simulink subsystem "Aerodyn"  (R2020b)
settings: Solver=VariableStepAuto  StartTime=0.0  StopTime=10.0  RelTol=1e-3
undefined symbols (not defined in the file or in its folder): Aerodynamics
settings Model: Creator=NicolasS  LastModifiedBy=leifr

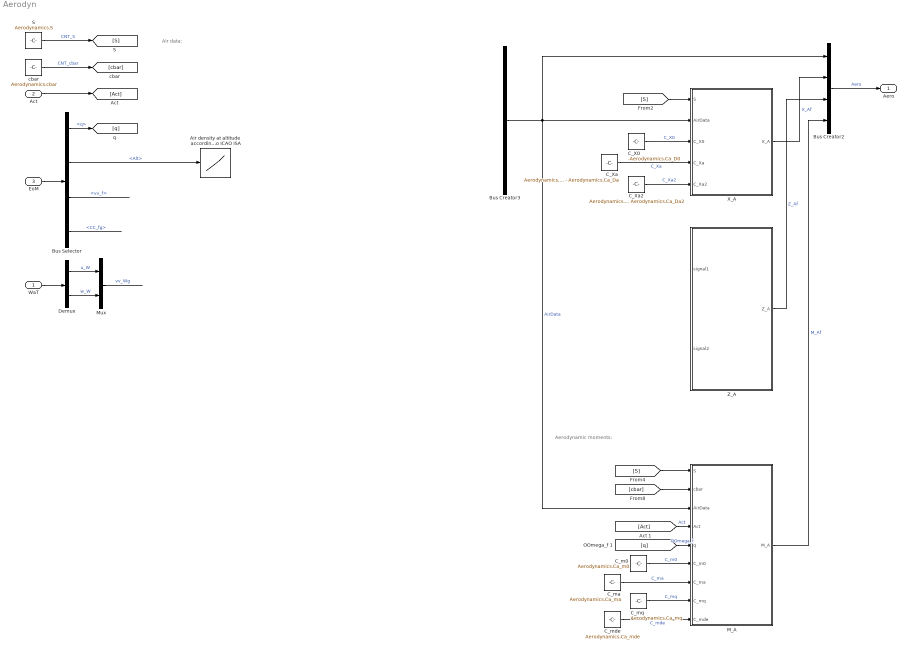
== system Aerodyn ==
  note: Aerodynamic moments:
  note: Air data:
  WaT : Inport
  Act : Inport  Port=2  OutDataTypeStr=Bus: Act
  EoM : Inport  Port=3  OutDataTypeStr=Bus: EoM
  Air density at altitude according to ICAO ISA : Lookup_n-D  NumberOfTableDimensions=1  BreakpointsForDimension1=Aerodynamics.LUT_Alt  Table=Aerodynamics.LUT_rho  ExtrapMethod=Clip  InternalRulePriority=Speed  RndMeth=Simplest  InputSameDT=on
  Bus Creator2 : BusCreator  Inputs=4  OutDataTypeStr=Bus: Aero
  Bus Creator3 : BusCreator  Inputs=5  OutDataTypeStr=Bus: AirData
  Bus Selector : BusSelector  OutputSignals=q,Alt,vv_f,CC.CC_fg
  C_X0 : Constant  Value=-Aerodynamics.Ca_D0  VectorParams1D=off  OutDataTypeStr=double  SampleTime=-1
  C_Xa : Constant  Value=Aerodynamics.Ca_L0 - Aerodynamics.Ca_Da  VectorParams1D=off  OutDataTypeStr=double  SampleTime=-1
  C_Xa2 : Constant  Value=Aerodynamics.Ca_La - Aerodynamics.Ca_Da2  VectorParams1D=off  OutDataTypeStr=double  SampleTime=-1
  C_m0 : Constant  Value=Aerodynamics.Ca_m0  VectorParams1D=off  OutDataTypeStr=double  SampleTime=-1
  C_ma : Constant  Value=Aerodynamics.Ca_ma  VectorParams1D=off  OutDataTypeStr=double  SampleTime=-1
  C_mde : Constant  Value=Aerodynamics.Ca_mde  VectorParams1D=off  OutDataTypeStr=double  SampleTime=-1
  C_mq : Constant  Value=Aerodynamics.Ca_mq  VectorParams1D=off  OutDataTypeStr=double  SampleTime=-1
  Demux : Demux  Outputs=2
  M_A : MATLAB Function  TreatAsAtomicUnit=on
  Mux : Mux  Inputs=2
  S : Constant  Value=Aerodynamics.S  OutDataTypeStr=double  SampleTime=-1
  X_A : MATLAB Function  TreatAsAtomicUnit=on
  Z_A : MATLAB Function  TreatAsAtomicUnit=on
  cbar : Constant  Value=Aerodynamics.cbar  OutDataTypeStr=double  SampleTime=-1
  Aero : Outport  OutDataTypeStr=Bus: Aero
  wires:
  C_m0/1 -> M_A/6(C_m0)  "C_m0"
  Bus Selector/4 -> ?  "<CC_fg>"
  ? -> Bus Creator3/1  "u_Af"
  Bus Creator2/1 -> Aero/1  "Aero"
  C_mde/1 -> M_A/9(C_mde)  "C_mde"
  S/1 -> [S]  "CNT_S"
  C_Xa/1 -> X_A/4(C_Xa)  "C_Xa"
  Bus Creator3/1 -> X_A/2(AirData), M_A/3(AirData), Bus Creator2/1  "AirData"
  EoM/1 -> Bus Selector/1
  M_A/1(M_A) -> Bus Creator2/4  "M_Af"
  Z_A/1(Z_A) -> Bus Creator2/3  "Z_Af"
  ? -> Bus Creator3/2  "w_Af"
  C_ma/1 -> M_A/7(C_ma)  "C_ma"
  C_mq/1 -> M_A/8(C_mq)  "C_mq"
  X_A/1(X_A) -> Bus Creator2/2  "X_Af"
  C_X0/1 -> X_A/3(C_X0)  "C_X0"
  [S] -> M_A/1(S)
  [q] -> M_A/5(q)  "OOmega_f"
  ? -> Bus Creator3/4  "p_dyn"
  [Act] -> M_A/4(Act)  "Act"
  Demux/2 -> Mux/2  "w_W"
  [cbar] -> M_A/2(cbar)
  Bus Selector/2 -> Air density at altitude according to ICAO ISA/1  "<Alt>"
  C_Xa2/1 -> X_A/5(C_Xa2)  "C_Xa2"
  WaT/1 -> Demux/1
  cbar/1 -> [cbar]  "CNT_cbar"
  Bus Selector/1 -> [q]  "<q>"
  Mux/1 -> ?  "vv_Wg"
  Demux/1 -> Mux/1  "u_W"
  Act/1 -> [Act]
  ? -> Bus Creator3/3  "V_A"
  [S] -> X_A/1(S)
  ? -> Bus Creator3/5  "alpha"
  Bus Selector/3 -> ?  "<vv_f>"

== matlab function Aerodyn/Z_A ==
  data: signal1 input; signal2 input; Z_A output

%%%%%%%%%%%%%%%%%%%%%%
% Body-fixed Z force %
%%%%%%%%%%%%%%%%%%%%%%

function Z_A = fcn(signal1, signal2)

Z_A = AirData.p_dyn*S*0;

== matlab function Aerodyn/M_A ==
  data: S input; cbar input; AirData input Bus: AirData size=1; Act input; q input; C_m0 input; C_ma input; C_mq input; C_mde input; M_A output

%%%%%%%%%%%%%%%%%%%%%%%%%%%
% Body-fixed pitch moment %
%%%%%%%%%%%%%%%%%%%%%%%%%%%

function M_A = fcn(S,cbar,AirData,Act,q,C_m0,C_ma,C_mq,C_mde)

M_A = AirData.p_dyn*S*cbar*(C_m0 + ...
                            0 + ...
                            0 + ...
                            0);

== matlab function Aerodyn/X_A ==
  data: S input; AirData input Bus: AirData size=1; C_X0 input; C_Xa input; C_Xa2 input; X_A output

%%%%%%%%%%%%%%%%%%%%%%
% Body-fixed X force %
%%%%%%%%%%%%%%%%%%%%%%

function X_A = fcn(S,AirData,C_X0,C_Xa,C_Xa2)

X_A = AirData.p_dyn*S*(C_X0 + ...
                       0 + ...
                      0);
